simulink model "C_TrigSubsysDialog"  (R2019b)
settings: Solver=ode45  StartTime=0.0  StopTime=10  RelTol=1e-3  EnableMultiTasking=on
model workspace (MAT data in the model file):
  AFS = 30
  AS = 0.5
  DT = 5
  cw = 1.3
  g = 9.81
  h0 = 500
  h1 = 150
  m = 85
  rho = 1.2
  v0 = 0
settings Model: Creator=Reichl  LastModifiedBy=jakob
settings DataIOCC: SaveFormat=Array  ReturnWorkspaceOutputs=off  OutputSaveName=h
settings OptimizationCC: LifeSpan=inf
settings DebuggingCC: SolverPrmCheckMsg=warning  SFUnexpectedBacktrackingDiag=warning  SFNoUnconditionalDefaultTransitionDiag=warning  SFExecutionAtInitializationDiag=none  ArithmeticOperatorsInVariantConditions=warning
settings HardwareCC: ProdBitPerPointer=32  ProdBitPerSizeT=32  ProdBitPerPtrDiffT=32  ProdLargestAtomicFloat=None  ProdIntDivRoundTo=Undefined  ProdEndianess=Unspecified  ProdWordSize=32  ProdHWDeviceType=32-bit Generic
settings ModelReferenceCC: PropagateSignalLabelsOutOfModel=off
settings SFSimCC: SimUseLocalCustomCode=off  CustomCodeUndefinedFunction=UseInterfaceOnly
settings RTWCC: RTWUseLocalCustomCode=off
settings CodeAppCC: StateflowObjectComments=on
settings GRTTargetCC: TargetLangStandard=C89/C90 (ANSI)  GeneratePreprocessorConditionals=Disable all
settings ConfigComp: CovMetricSettings=dw  CovHtmlReporting=on  CovSaveCumulativeToWorkspaceVar=on  CovSaveSingleToWorkspaceVar=on  CovExternalEMLEnable=off  CovSFcnEnable=off

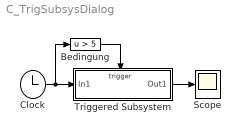
== system C_TrigSubsysDialog ==
  Bedingung : Fcn  Expr=u > 5
  Clock : Clock
  Scope : Scope
  Triggered Subsystem : Subsystem  TreatAsAtomicUnit=on
  wires:
  Clock/1 -> Bedingung/1, Triggered Subsystem/1(In1)
  Bedingung/1 -> Triggered Subsystem/Trigger
  Triggered Subsystem/1(Out1) -> Scope/1

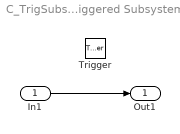
== system C_TrigSubsysDialog/Triggered Subsystem ==
  In1 : Inport
  Trigger : TriggerPort  VariantControl=Variant
  Out1 : Outport  InitialOutput=1.5  VectorParamsAs1DForOutWhenUnconnected=off
  wires:
  In1/1 -> Out1/1
